simulink model "SchmittTrigger_mod"  (Simulink 8.1)
settings: Solver=FixedStepDiscrete  StartTime=0.0  StopTime=1/20*2  FixedStep=1/(20*100)  RelTol=1e-3
values from neighbouring files (symbols this model uses):
  A = 5    [SchmittTrigger_data.m]    (also in Uebung2.m = 3; Uebung5.m = 3; Uebung6_2.m = zeros(1,N+1))
  f = 20    [SchmittTrigger_data.m]    (also in Uebung1.m = [e e e e e]; Uebung2.m = 1000; Uebung6_1.m = 0:fs/Nfft:fs/2; VL1_1St.m = 3.14159265359)
  Ua = 5    [SchmittTrigger_data.m]
  Us = 1    [SchmittTrigger_data.m]
  Us1 = 1    [SchmittTrigger_data.m]
settings Model: Creator=Uli  LastModifiedBy=Uli
settings OptimizationCC: BooleanDataType=off  ExpressionDepthLimit=128  InitFltsAndDblsToZero=on
settings DebuggingCC: SaveWithParameterizedLinksMsg=none  SignalResolutionControl=TryResolveAllWithWarning  SolverPrmCheckMsg=none  MultiTaskDSMMsg=warning  MultiTaskCondExecSysMsg=none  StrictBusMsg=None
settings HardwareCC: TargetUnknown=on
settings RTWCC: IncludeERTFirstTime=on
settings GRTTargetCC: TargetFcnLib=ansi_tfl_tmw.mat  ModelReferenceCompliant=off  MatFileLogging=off

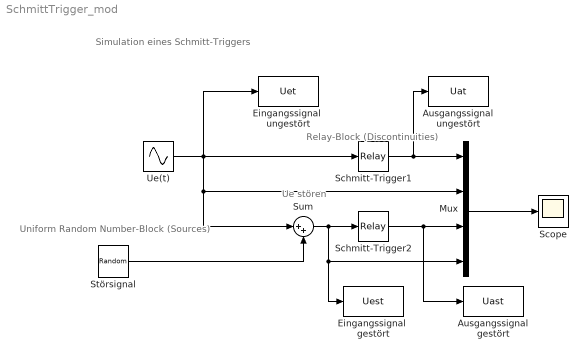
== system SchmittTrigger_mod ==
  note: Simulation eines Schmitt-Triggers
  note: Ue stören
  note: Relay-Block
      | (Discontinuities)
  note: Uniform Random Number-Block
      | (Sources)
  Ausgangssignal gestört : ToWorkspace  VariableName=Uast  SampleTime=-1
  Ausgangssignal ungestört : ToWorkspace  VariableName=Uat  SampleTime=-1
  Eingangssignal  gestört : ToWorkspace  VariableName=Uest  SampleTime=-1
  Eingangssignal  ungestört : ToWorkspace  VariableName=Uet  SampleTime=-1
  Mux : Mux
  Schmitt-Trigger1 : Relay  OnSwitchValue=Us  OffSwitchValue=-Us  OnOutputValue=Ua  OffOutputValue=-Ua
  Schmitt-Trigger2 : Relay  OnSwitchValue=Us1  OffSwitchValue=-Us1  OnOutputValue=Ua  OffOutputValue=-Ua
  Scope : Scope
  Störsignal : UniformRandomNumber  Minimum=-3  Maximum=3  SampleTime=0
  Sum : Sum  Inputs=|++  SaturateOnIntegerOverflow=on  InputSameDT=on  OutDataTypeStr=Inherit: Same as first input
  Ue(t) : Sin  Amplitude=A  Frequency=2*pi*f  SampleTime=0
  wires:
  Ue(t)/1 -> Sum/1, Mux/2, Schmitt-Trigger1/1, Eingangssignal  ungestört/1
  Schmitt-Trigger1/1 -> Mux/1, Ausgangssignal ungestört/1
  Mux/1 -> Scope/1
  Störsignal/1 -> Sum/2
  Sum/1 -> Schmitt-Trigger2/1, Mux/4, Eingangssignal  gestört/1
  Schmitt-Trigger2/1 -> Mux/3, Ausgangssignal gestört/1
